simulink library "FG_Controller_Library"  (R2017b)
settings: Solver=VariableStepAuto  StartTime=0.0  StopTime=10.0  RelTol=1e-3
undefined symbols (not defined in the file or in its folder): fcut_velocity_joint, GaitLibrary, isSim, UserParams
libraries: slrtlib x113, simulink x1, func_block_library x1
(part 2 of 3)

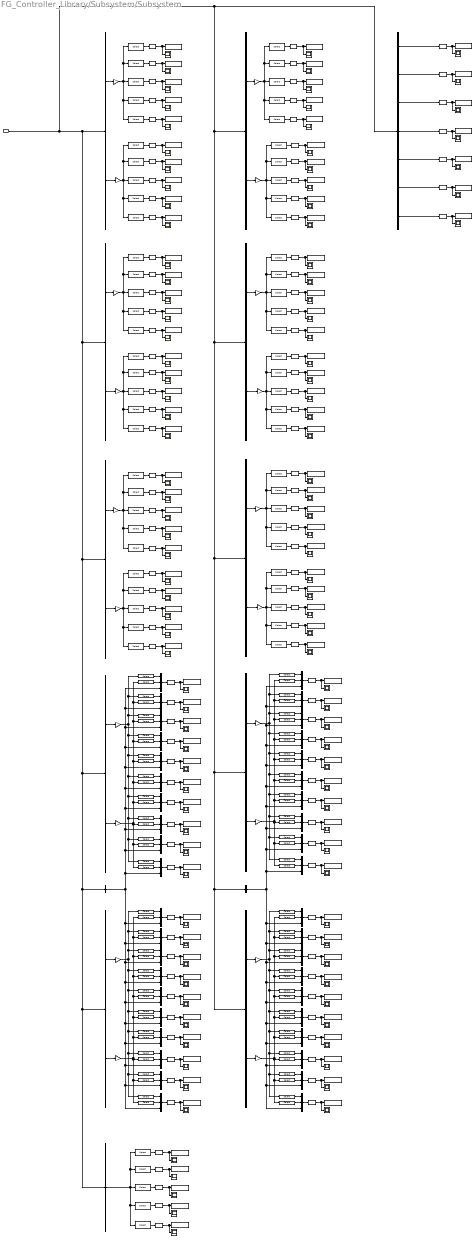
== system FG_Controller_Library/Subsystem/Subsystem ==
  In1 : Inport  OutDataTypeStr=Bus: cassieDataBus
  Bus Selector : BusSelector  OutputSignals=hd,dhd
  Bus Selector1 : BusSelector  OutputSignals=hd_joint,dhd_joint
  Bus Selector10 : BusSelector  OutputSignals=dh0_joint,dhd_joint
  Bus Selector11 : BusSelector  OutputSignals=stanceLeg
  Bus Selector12 : BusSelector  OutputSignals=u
  Bus Selector13 : BusSelector  OutputSignals=torso_vx_b,torso_vy_b,torso_vz_b,torso_vx_b_fil,torso_vy_b_fil,torso_vz_b_fil,tg_velocity_x
  Bus Selector2 : BusSelector  OutputSignals=h0,dh0
  Bus Selector3 : BusSelector  OutputSignals=h0_joint,dh0_joint
  Bus Selector4 : BusSelector  OutputSignals=y,dy
  Bus Selector5 : BusSelector  OutputSignals=y_joint,dy_joint
  Bus Selector6 : BusSelector  OutputSignals=hd,h0
  Bus Selector7 : BusSelector  OutputSignals=stanceLeg
  Bus Selector8 : BusSelector  OutputSignals=hd_joint,h0_joint
  Bus Selector9 : BusSelector  OutputSignals=dhd,dh0
  Gain{,1..19} (20 alike) : Gain  Gain=180/pi
  Mux{,1..39} (40 alike) : Mux  Inputs=3
  Reshape{,1..111} (112 alike) : Reshape
  Scope{,1..111} (112 alike) : Scope
  "Scope " : slrtlib/Displays and Logging/Scope   scopeno=201  scopetype=Host  autostart=on  viewmode=Graphical redraw  formatstr='%15.6f'  grid=on  ylimits=[0,0]  nosamples=2500  noprepostsamples=0  interleave=1  triggermode=FreeRun  triggersignal=1  trigsignalfromport=off  triggerlevel=0.0  triggerslope=Either  triggerscope=1  triggersample=0  filename=data.dat  mode=Lazy  writesize=512  autorestart=off  dynamicfilemode=off  maxwritefilesize=512*1024^2
  Scope 1 : slrtlib/Displays and Logging/Scope   scopeno=202  scopetype=Host  autostart=on  viewmode=Graphical redraw  formatstr='%15.6f'  grid=on  ylimits=[0,0]  nosamples=2500  noprepostsamples=0  interleave=1  triggermode=FreeRun  triggersignal=1  trigsignalfromport=off  triggerlevel=0.0  triggerslope=Either  triggerscope=1  triggersample=0  filename=data.dat  mode=Lazy  writesize=512  autorestart=off  dynamicfilemode=off  maxwritefilesize=512*1024^2
  Scope 10 : slrtlib/Displays and Logging/Scope   scopeno=2201  scopetype=Host  autostart=on  viewmode=Graphical redraw  formatstr='%15.6f'  grid=on  ylimits=[0,0]  nosamples=2500  noprepostsamples=0  interleave=1  triggermode=FreeRun  triggersignal=1  trigsignalfromport=off  triggerlevel=0.0  triggerslope=Either  triggerscope=1  triggersample=0  filename=data.dat  mode=Lazy  writesize=512  autorestart=off  dynamicfilemode=off  maxwritefilesize=512*1024^2
  Scope 100 : slrtlib/Displays and Logging/Scope   scopeno=701  scopetype=Host  autostart=on  viewmode=Graphical redraw  formatstr='%15.6f'  grid=on  ylimits=[0,0]  nosamples=2500  noprepostsamples=0  interleave=1  triggermode=FreeRun  triggersignal=1  trigsignalfromport=off  triggerlevel=0.0  triggerslope=Either  triggerscope=1  triggersample=0  filename=data.dat  mode=Lazy  writesize=512  autorestart=off  dynamicfilemode=off  maxwritefilesize=512*1024^2
  Scope 101 : slrtlib/Displays and Logging/Scope   scopeno=702  scopetype=Host  autostart=on  viewmode=Graphical redraw  formatstr='%15.6f'  grid=on  ylimits=[0,0]  nosamples=2500  noprepostsamples=0  interleave=1  triggermode=FreeRun  triggersignal=1  trigsignalfromport=off  triggerlevel=0.0  triggerslope=Either  triggerscope=1  triggersample=0  filename=data.dat  mode=Lazy  writesize=512  autorestart=off  dynamicfilemode=off  maxwritefilesize=512*1024^2
  Scope 102 : slrtlib/Displays and Logging/Scope   scopeno=703  scopetype=Host  autostart=on  viewmode=Graphical redraw  formatstr='%15.6f'  grid=on  ylimits=[0,0]  nosamples=2500  noprepostsamples=0  interleave=1  triggermode=FreeRun  triggersignal=1  trigsignalfromport=off  triggerlevel=0.0  triggerslope=Either  triggerscope=1  triggersample=0  filename=data.dat  mode=Lazy  writesize=512  autorestart=off  dynamicfilemode=off  maxwritefilesize=512*1024^2
  Scope 103 : slrtlib/Displays and Logging/Scope   scopeno=704  scopetype=Host  autostart=on  viewmode=Graphical redraw  formatstr='%15.6f'  grid=on  ylimits=[0,0]  nosamples=2500  noprepostsamples=0  interleave=1  triggermode=FreeRun  triggersignal=1  trigsignalfromport=off  triggerlevel=0.0  triggerslope=Either  triggerscope=1  triggersample=0  filename=data.dat  mode=Lazy  writesize=512  autorestart=off  dynamicfilemode=off  maxwritefilesize=512*1024^2
  Scope 104 : slrtlib/Displays and Logging/Scope   scopeno=705  scopetype=Host  autostart=on  viewmode=Graphical redraw  formatstr='%15.6f'  grid=on  ylimits=[0,0]  nosamples=2500  noprepostsamples=0  interleave=1  triggermode=FreeRun  triggersignal=1  trigsignalfromport=off  triggerlevel=0.0  triggerslope=Either  triggerscope=1  triggersample=0  filename=data.dat  mode=Lazy  writesize=512  autorestart=off  dynamicfilemode=off  maxwritefilesize=512*1024^2
  Scope 105 : slrtlib/Displays and Logging/Scope   scopeno=901  scopetype=Host  autostart=on  viewmode=Graphical redraw  formatstr='%15.6f'  grid=on  ylimits=[0,0]  nosamples=2500  noprepostsamples=0  interleave=1  triggermode=FreeRun  triggersignal=1  trigsignalfromport=off  triggerlevel=0.0  triggerslope=Either  triggerscope=1  triggersample=0  filename=data.dat  mode=Lazy  writesize=512  autorestart=off  dynamicfilemode=off  maxwritefilesize=512*1024^2
  Scope 106 : slrtlib/Displays and Logging/Scope   scopeno=902  scopetype=Host  autostart=on  viewmode=Graphical redraw  formatstr='%15.6f'  grid=on  ylimits=[0,0]  nosamples=2500  noprepostsamples=0  interleave=1  triggermode=FreeRun  triggersignal=1  trigsignalfromport=off  triggerlevel=0.0  triggerslope=Either  triggerscope=1  triggersample=0  filename=data.dat  mode=Lazy  writesize=512  autorestart=off  dynamicfilemode=off  maxwritefilesize=512*1024^2
  Scope 107 : slrtlib/Displays and Logging/Scope   scopeno=903  scopetype=Host  autostart=on  viewmode=Graphical redraw  formatstr='%15.6f'  grid=on  ylimits=[0,0]  nosamples=2500  noprepostsamples=0  interleave=1  triggermode=FreeRun  triggersignal=1  trigsignalfromport=off  triggerlevel=0.0  triggerslope=Either  triggerscope=1  triggersample=0  filename=data.dat  mode=Lazy  writesize=512  autorestart=off  dynamicfilemode=off  maxwritefilesize=512*1024^2
  Scope 108 : slrtlib/Displays and Logging/Scope   scopeno=904  scopetype=Host  autostart=on  viewmode=Graphical redraw  formatstr='%15.6f'  grid=on  ylimits=[0,0]  nosamples=2500  noprepostsamples=0  interleave=1  triggermode=FreeRun  triggersignal=1  trigsignalfromport=off  triggerlevel=0.0  triggerslope=Either  triggerscope=1  triggersample=0  filename=data.dat  mode=Lazy  writesize=512  autorestart=off  dynamicfilemode=off  maxwritefilesize=512*1024^2
  Scope 109 : slrtlib/Displays and Logging/Scope   scopeno=905  scopetype=Host  autostart=on  viewmode=Graphical redraw  formatstr='%15.6f'  grid=on  ylimits=[0,0]  nosamples=2500  noprepostsamples=0  interleave=1  triggermode=FreeRun  triggersignal=1  trigsignalfromport=off  triggerlevel=0.0  triggerslope=Either  triggerscope=1  triggersample=0  filename=data.dat  mode=Lazy  writesize=512  autorestart=off  dynamicfilemode=off  maxwritefilesize=512*1024^2
  Scope 11 : slrtlib/Displays and Logging/Scope   scopeno=2202  scopetype=Host  autostart=on  viewmode=Graphical redraw  formatstr='%15.6f'  grid=on  ylimits=[0,0]  nosamples=2500  noprepostsamples=0  interleave=1  triggermode=FreeRun  triggersignal=1  trigsignalfromport=off  triggerlevel=0.0  triggerslope=Either  triggerscope=1  triggersample=0  filename=data.dat  mode=Lazy  writesize=512  autorestart=off  dynamicfilemode=off  maxwritefilesize=512*1024^2
  Scope 110 : slrtlib/Displays and Logging/Scope   scopeno=906  scopetype=Host  autostart=on  viewmode=Graphical redraw  formatstr='%15.6f'  grid=on  ylimits=[0,0]  nosamples=2500  noprepostsamples=0  interleave=1  triggermode=FreeRun  triggersignal=1  trigsignalfromport=off  triggerlevel=0.0  triggerslope=Either  triggerscope=1  triggersample=0  filename=data.dat  mode=Lazy  writesize=512  autorestart=off  dynamicfilemode=off  maxwritefilesize=512*1024^2
  Scope 111 : slrtlib/Displays and Logging/Scope   scopeno=907  scopetype=Host  autostart=on  viewmode=Graphical redraw  formatstr='%15.6f'  grid=on  ylimits=[0,0]  nosamples=2500  noprepostsamples=0  interleave=1  triggermode=FreeRun  triggersignal=1  trigsignalfromport=off  triggerlevel=0.0  triggerslope=Either  triggerscope=1  triggersample=0  filename=data.dat  mode=Lazy  writesize=512  autorestart=off  dynamicfilemode=off  maxwritefilesize=512*1024^2
  Scope 12 : slrtlib/Displays and Logging/Scope   scopeno=2203  scopetype=Host  autostart=on  viewmode=Graphical redraw  formatstr='%15.6f'  grid=on  ylimits=[0,0]  nosamples=2500  noprepostsamples=0  interleave=1  triggermode=FreeRun  triggersignal=1  trigsignalfromport=off  triggerlevel=0.0  triggerslope=Either  triggerscope=1  triggersample=0  filename=data.dat  mode=Lazy  writesize=512  autorestart=off  dynamicfilemode=off  maxwritefilesize=512*1024^2
  Scope 13 : slrtlib/Displays and Logging/Scope   scopeno=2204  scopetype=Host  autostart=on  viewmode=Graphical redraw  formatstr='%15.6f'  grid=on  ylimits=[0,0]  nosamples=2500  noprepostsamples=0  interleave=1  triggermode=FreeRun  triggersignal=1  trigsignalfromport=off  triggerlevel=0.0  triggerslope=Either  triggerscope=1  triggersample=0  filename=data.dat  mode=Lazy  writesize=512  autorestart=off  dynamicfilemode=off  maxwritefilesize=512*1024^2
  Scope 14 : slrtlib/Displays and Logging/Scope   scopeno=2205  scopetype=Host  autostart=on  viewmode=Graphical redraw  formatstr='%15.6f'  grid=on  ylimits=[0,0]  nosamples=2500  noprepostsamples=0  interleave=1  triggermode=FreeRun  triggersignal=1  trigsignalfromport=off  triggerlevel=0.0  triggerslope=Either  triggerscope=1  triggersample=0  filename=data.dat  mode=Lazy  writesize=512  autorestart=off  dynamicfilemode=off  maxwritefilesize=512*1024^2
  Scope 15 : slrtlib/Displays and Logging/Scope   scopeno=2206  scopetype=Host  autostart=on  viewmode=Graphical redraw  formatstr='%15.6f'  grid=on  ylimits=[0,0]  nosamples=2500  noprepostsamples=0  interleave=1  triggermode=FreeRun  triggersignal=1  trigsignalfromport=off  triggerlevel=0.0  triggerslope=Either  triggerscope=1  triggersample=0  filename=data.dat  mode=Lazy  writesize=512  autorestart=off  dynamicfilemode=off  maxwritefilesize=512*1024^2
  Scope 16 : slrtlib/Displays and Logging/Scope   scopeno=2207  scopetype=Host  autostart=on  viewmode=Graphical redraw  formatstr='%15.6f'  grid=on  ylimits=[0,0]  nosamples=2500  noprepostsamples=0  interleave=1  triggermode=FreeRun  triggersignal=1  trigsignalfromport=off  triggerlevel=0.0  triggerslope=Either  triggerscope=1  triggersample=0  filename=data.dat  mode=Lazy  writesize=512  autorestart=off  dynamicfilemode=off  maxwritefilesize=512*1024^2
  Scope 17 : slrtlib/Displays and Logging/Scope   scopeno=2208  scopetype=Host  autostart=on  viewmode=Graphical redraw  formatstr='%15.6f'  grid=on  ylimits=[0,0]  nosamples=2500  noprepostsamples=0  interleave=1  triggermode=FreeRun  triggersignal=1  trigsignalfromport=off  triggerlevel=0.0  triggerslope=Either  triggerscope=1  triggersample=0  filename=data.dat  mode=Lazy  writesize=512  autorestart=off  dynamicfilemode=off  maxwritefilesize=512*1024^2
  Scope 18 : slrtlib/Displays and Logging/Scope   scopeno=2209  scopetype=Host  autostart=on  viewmode=Graphical redraw  formatstr='%15.6f'  grid=on  ylimits=[0,0]  nosamples=2500  noprepostsamples=0  interleave=1  triggermode=FreeRun  triggersignal=1  trigsignalfromport=off  triggerlevel=0.0  triggerslope=Either  triggerscope=1  triggersample=0  filename=data.dat  mode=Lazy  writesize=512  autorestart=off  dynamicfilemode=off  maxwritefilesize=512*1024^2
  Scope 19 : slrtlib/Displays and Logging/Scope   scopeno=2210  scopetype=Host  autostart=on  viewmode=Graphical redraw  formatstr='%15.6f'  grid=on  ylimits=[0,0]  nosamples=2500  noprepostsamples=0  interleave=1  triggermode=FreeRun  triggersignal=1  trigsignalfromport=off  triggerlevel=0.0  triggerslope=Either  triggerscope=1  triggersample=0  filename=data.dat  mode=Lazy  writesize=512  autorestart=off  dynamicfilemode=off  maxwritefilesize=512*1024^2
  Scope 2 : slrtlib/Displays and Logging/Scope   scopeno=203  scopetype=Host  autostart=on  viewmode=Graphical redraw  formatstr='%15.6f'  grid=on  ylimits=[0,0]  nosamples=2500  noprepostsamples=0  interleave=1  triggermode=FreeRun  triggersignal=1  trigsignalfromport=off  triggerlevel=0.0  triggerslope=Either  triggerscope=1  triggersample=0  filename=data.dat  mode=Lazy  writesize=512  autorestart=off  dynamicfilemode=off  maxwritefilesize=512*1024^2
  Scope 20 : slrtlib/Displays and Logging/Scope   scopeno=301  scopetype=Host  autostart=on  viewmode=Graphical redraw  formatstr='%15.6f'  grid=on  ylimits=[0,0]  nosamples=2500  noprepostsamples=0  interleave=1  triggermode=FreeRun  triggersignal=1  trigsignalfromport=off  triggerlevel=0.0  triggerslope=Either  triggerscope=1  triggersample=0  filename=data.dat  mode=Lazy  writesize=512  autorestart=off  dynamicfilemode=off  maxwritefilesize=512*1024^2
  Scope 21 : slrtlib/Displays and Logging/Scope   scopeno=302  scopetype=Host  autostart=on  viewmode=Graphical redraw  formatstr='%15.6f'  grid=on  ylimits=[0,0]  nosamples=2500  noprepostsamples=0  interleave=1  triggermode=FreeRun  triggersignal=1  trigsignalfromport=off  triggerlevel=0.0  triggerslope=Either  triggerscope=1  triggersample=0  filename=data.dat  mode=Lazy  writesize=512  autorestart=off  dynamicfilemode=off  maxwritefilesize=512*1024^2
  Scope 22 : slrtlib/Displays and Logging/Scope   scopeno=303  scopetype=Host  autostart=on  viewmode=Graphical redraw  formatstr='%15.6f'  grid=on  ylimits=[0,0]  nosamples=2500  noprepostsamples=0  interleave=1  triggermode=FreeRun  triggersignal=1  trigsignalfromport=off  triggerlevel=0.0  triggerslope=Either  triggerscope=1  triggersample=0  filename=data.dat  mode=Lazy  writesize=512  autorestart=off  dynamicfilemode=off  maxwritefilesize=512*1024^2
  Scope 23 : slrtlib/Displays and Logging/Scope   scopeno=304  scopetype=Host  autostart=on  viewmode=Graphical redraw  formatstr='%15.6f'  grid=on  ylimits=[0,0]  nosamples=2500  noprepostsamples=0  interleave=1  triggermode=FreeRun  triggersignal=1  trigsignalfromport=off  triggerlevel=0.0  triggerslope=Either  triggerscope=1  triggersample=0  filename=data.dat  mode=Lazy  writesize=512  autorestart=off  dynamicfilemode=off  maxwritefilesize=512*1024^2
  Scope 24 : slrtlib/Displays and Logging/Scope   scopeno=305  scopetype=Host  autostart=on  viewmode=Graphical redraw  formatstr='%15.6f'  grid=on  ylimits=[0,0]  nosamples=2500  noprepostsamples=0  interleave=1  triggermode=FreeRun  triggersignal=1  trigsignalfromport=off  triggerlevel=0.0  triggerslope=Either  triggerscope=1  triggersample=0  filename=data.dat  mode=Lazy  writesize=512  autorestart=off  dynamicfilemode=off  maxwritefilesize=512*1024^2
  Scope 25 : slrtlib/Displays and Logging/Scope   scopeno=306  scopetype=Host  autostart=on  viewmode=Graphical redraw  formatstr='%15.6f'  grid=on  ylimits=[0,0]  nosamples=2500  noprepostsamples=0  interleave=1  triggermode=FreeRun  triggersignal=1  trigsignalfromport=off  triggerlevel=0.0  triggerslope=Either  triggerscope=1  triggersample=0  filename=data.dat  mode=Lazy  writesize=512  autorestart=off  dynamicfilemode=off  maxwritefilesize=512*1024^2
  Scope 26 : slrtlib/Displays and Logging/Scope   scopeno=307  scopetype=Host  autostart=on  viewmode=Graphical redraw  formatstr='%15.6f'  grid=on  ylimits=[0,0]  nosamples=2500  noprepostsamples=0  interleave=1  triggermode=FreeRun  triggersignal=1  trigsignalfromport=off  triggerlevel=0.0  triggerslope=Either  triggerscope=1  triggersample=0  filename=data.dat  mode=Lazy  writesize=512  autorestart=off  dynamicfilemode=off  maxwritefilesize=512*1024^2
  Scope 27 : slrtlib/Displays and Logging/Scope   scopeno=308  scopetype=Host  autostart=on  viewmode=Graphical redraw  formatstr='%15.6f'  grid=on  ylimits=[0,0]  nosamples=2500  noprepostsamples=0  interleave=1  triggermode=FreeRun  triggersignal=1  trigsignalfromport=off  triggerlevel=0.0  triggerslope=Either  triggerscope=1  triggersample=0  filename=data.dat  mode=Lazy  writesize=512  autorestart=off  dynamicfilemode=off  maxwritefilesize=512*1024^2
  Scope 28 : slrtlib/Displays and Logging/Scope   scopeno=309  scopetype=Host  autostart=on  viewmode=Graphical redraw  formatstr='%15.6f'  grid=on  ylimits=[0,0]  nosamples=2500  noprepostsamples=0  interleave=1  triggermode=FreeRun  triggersignal=1  trigsignalfromport=off  triggerlevel=0.0  triggerslope=Either  triggerscope=1  triggersample=0  filename=data.dat  mode=Lazy  writesize=512  autorestart=off  dynamicfilemode=off  maxwritefilesize=512*1024^2
  Scope 29 : slrtlib/Displays and Logging/Scope   scopeno=310  scopetype=Host  autostart=on  viewmode=Graphical redraw  formatstr='%15.6f'  grid=on  ylimits=[0,0]  nosamples=2500  noprepostsamples=0  interleave=1  triggermode=FreeRun  triggersignal=1  trigsignalfromport=off  triggerlevel=0.0  triggerslope=Either  triggerscope=1  triggersample=0  filename=data.dat  mode=Lazy  writesize=512  autorestart=off  dynamicfilemode=off  maxwritefilesize=512*1024^2
  Scope 3 : slrtlib/Displays and Logging/Scope   scopeno=204  scopetype=Host  autostart=on  viewmode=Graphical redraw  formatstr='%15.6f'  grid=on  ylimits=[0,0]  nosamples=2500  noprepostsamples=0  interleave=1  triggermode=FreeRun  triggersignal=1  trigsignalfromport=off  triggerlevel=0.0  triggerslope=Either  triggerscope=1  triggersample=0  filename=data.dat  mode=Lazy  writesize=512  autorestart=off  dynamicfilemode=off  maxwritefilesize=512*1024^2
  Scope 30 : slrtlib/Displays and Logging/Scope   scopeno=3301  scopetype=Host  autostart=on  viewmode=Graphical redraw  formatstr='%15.6f'  grid=on  ylimits=[0,0]  nosamples=2500  noprepostsamples=0  interleave=1  triggermode=FreeRun  triggersignal=1  trigsignalfromport=off  triggerlevel=0.0  triggerslope=Either  triggerscope=1  triggersample=0  filename=data.dat  mode=Lazy  writesize=512  autorestart=off  dynamicfilemode=off  maxwritefilesize=512*1024^2
  Scope 31 : slrtlib/Displays and Logging/Scope   scopeno=3302  scopetype=Host  autostart=on  viewmode=Graphical redraw  formatstr='%15.6f'  grid=on  ylimits=[0,0]  nosamples=2500  noprepostsamples=0  interleave=1  triggermode=FreeRun  triggersignal=1  trigsignalfromport=off  triggerlevel=0.0  triggerslope=Either  triggerscope=1  triggersample=0  filename=data.dat  mode=Lazy  writesize=512  autorestart=off  dynamicfilemode=off  maxwritefilesize=512*1024^2
  Scope 32 : slrtlib/Displays and Logging/Scope   scopeno=3303  scopetype=Host  autostart=on  viewmode=Graphical redraw  formatstr='%15.6f'  grid=on  ylimits=[0,0]  nosamples=2500  noprepostsamples=0  interleave=1  triggermode=FreeRun  triggersignal=1  trigsignalfromport=off  triggerlevel=0.0  triggerslope=Either  triggerscope=1  triggersample=0  filename=data.dat  mode=Lazy  writesize=512  autorestart=off  dynamicfilemode=off  maxwritefilesize=512*1024^2
  Scope 33 : slrtlib/Displays and Logging/Scope   scopeno=3304  scopetype=Host  autostart=on  viewmode=Graphical redraw  formatstr='%15.6f'  grid=on  ylimits=[0,0]  nosamples=2500  noprepostsamples=0  interleave=1  triggermode=FreeRun  triggersignal=1  trigsignalfromport=off  triggerlevel=0.0  triggerslope=Either  triggerscope=1  triggersample=0  filename=data.dat  mode=Lazy  writesize=512  autorestart=off  dynamicfilemode=off  maxwritefilesize=512*1024^2
  Scope 34 : slrtlib/Displays and Logging/Scope   scopeno=3305  scopetype=Host  autostart=on  viewmode=Graphical redraw  formatstr='%15.6f'  grid=on  ylimits=[0,0]  nosamples=2500  noprepostsamples=0  interleave=1  triggermode=FreeRun  triggersignal=1  trigsignalfromport=off  triggerlevel=0.0  triggerslope=Either  triggerscope=1  triggersample=0  filename=data.dat  mode=Lazy  writesize=512  autorestart=off  dynamicfilemode=off  maxwritefilesize=512*1024^2
  Scope 35 : slrtlib/Displays and Logging/Scope   scopeno=3306  scopetype=Host  autostart=on  viewmode=Graphical redraw  formatstr='%15.6f'  grid=on  ylimits=[0,0]  nosamples=2500  noprepostsamples=0  interleave=1  triggermode=FreeRun  triggersignal=1  trigsignalfromport=off  triggerlevel=0.0  triggerslope=Either  triggerscope=1  triggersample=0  filename=data.dat  mode=Lazy  writesize=512  autorestart=off  dynamicfilemode=off  maxwritefilesize=512*1024^2
  Scope 36 : slrtlib/Displays and Logging/Scope   scopeno=3307  scopetype=Host  autostart=on  viewmode=Graphical redraw  formatstr='%15.6f'  grid=on  ylimits=[0,0]  nosamples=2500  noprepostsamples=0  interleave=1  triggermode=FreeRun  triggersignal=1  trigsignalfromport=off  triggerlevel=0.0  triggerslope=Either  triggerscope=1  triggersample=0  filename=data.dat  mode=Lazy  writesize=512  autorestart=off  dynamicfilemode=off  maxwritefilesize=512*1024^2
  Scope 37 : slrtlib/Displays and Logging/Scope   scopeno=3308  scopetype=Host  autostart=on  viewmode=Graphical redraw  formatstr='%15.6f'  grid=on  ylimits=[0,0]  nosamples=2500  noprepostsamples=0  interleave=1  triggermode=FreeRun  triggersignal=1  trigsignalfromport=off  triggerlevel=0.0  triggerslope=Either  triggerscope=1  triggersample=0  filename=data.dat  mode=Lazy  writesize=512  autorestart=off  dynamicfilemode=off  maxwritefilesize=512*1024^2
  Scope 38 : slrtlib/Displays and Logging/Scope   scopeno=3309  scopetype=Host  autostart=on  viewmode=Graphical redraw  formatstr='%15.6f'  grid=on  ylimits=[0,0]  nosamples=2500  noprepostsamples=0  interleave=1  triggermode=FreeRun  triggersignal=1  trigsignalfromport=off  triggerlevel=0.0  triggerslope=Either  triggerscope=1  triggersample=0  filename=data.dat  mode=Lazy  writesize=512  autorestart=off  dynamicfilemode=off  maxwritefilesize=512*1024^2
  Scope 39 : slrtlib/Displays and Logging/Scope   scopeno=3310  scopetype=Host  autostart=on  viewmode=Graphical redraw  formatstr='%15.6f'  grid=on  ylimits=[0,0]  nosamples=2500  noprepostsamples=0  interleave=1  triggermode=FreeRun  triggersignal=1  trigsignalfromport=off  triggerlevel=0.0  triggerslope=Either  triggerscope=1  triggersample=0  filename=data.dat  mode=Lazy  writesize=512  autorestart=off  dynamicfilemode=off  maxwritefilesize=512*1024^2
  Scope 4 : slrtlib/Displays and Logging/Scope   scopeno=205  scopetype=Host  autostart=on  viewmode=Graphical redraw  formatstr='%15.6f'  grid=on  ylimits=[0,0]  nosamples=2500  noprepostsamples=0  interleave=1  triggermode=FreeRun  triggersignal=1  trigsignalfromport=off  triggerlevel=0.0  triggerslope=Either  triggerscope=1  triggersample=0  filename=data.dat  mode=Lazy  writesize=512  autorestart=off  dynamicfilemode=off  maxwritefilesize=512*1024^2
  Scope 40 : slrtlib/Displays and Logging/Scope   scopeno=401  scopetype=Host  autostart=on  viewmode=Graphical redraw  formatstr='%15.6f'  grid=on  ylimits=[0,0]  nosamples=2500  noprepostsamples=0  interleave=1  triggermode=FreeRun  triggersignal=1  trigsignalfromport=off  triggerlevel=0.0  triggerslope=Either  triggerscope=1  triggersample=0  filename=data.dat  mode=Lazy  writesize=512  autorestart=off  dynamicfilemode=off  maxwritefilesize=512*1024^2
  Scope 41 : slrtlib/Displays and Logging/Scope   scopeno=402  scopetype=Host  autostart=on  viewmode=Graphical redraw  formatstr='%15.6f'  grid=on  ylimits=[0,0]  nosamples=2500  noprepostsamples=0  interleave=1  triggermode=FreeRun  triggersignal=1  trigsignalfromport=off  triggerlevel=0.0  triggerslope=Either  triggerscope=1  triggersample=0  filename=data.dat  mode=Lazy  writesize=512  autorestart=off  dynamicfilemode=off  maxwritefilesize=512*1024^2
  Scope 42 : slrtlib/Displays and Logging/Scope   scopeno=403  scopetype=Host  autostart=on  viewmode=Graphical redraw  formatstr='%15.6f'  grid=on  ylimits=[0,0]  nosamples=2500  noprepostsamples=0  interleave=1  triggermode=FreeRun  triggersignal=1  trigsignalfromport=off  triggerlevel=0.0  triggerslope=Either  triggerscope=1  triggersample=0  filename=data.dat  mode=Lazy  writesize=512  autorestart=off  dynamicfilemode=off  maxwritefilesize=512*1024^2
  Scope 43 : slrtlib/Displays and Logging/Scope   scopeno=404  scopetype=Host  autostart=on  viewmode=Graphical redraw  formatstr='%15.6f'  grid=on  ylimits=[0,0]  nosamples=2500  noprepostsamples=0  interleave=1  triggermode=FreeRun  triggersignal=1  trigsignalfromport=off  triggerlevel=0.0  triggerslope=Either  triggerscope=1  triggersample=0  filename=data.dat  mode=Lazy  writesize=512  autorestart=off  dynamicfilemode=off  maxwritefilesize=512*1024^2
  Scope 44 : slrtlib/Displays and Logging/Scope   scopeno=405  scopetype=Host  autostart=on  viewmode=Graphical redraw  formatstr='%15.6f'  grid=on  ylimits=[0,0]  nosamples=2500  noprepostsamples=0  interleave=1  triggermode=FreeRun  triggersignal=1  trigsignalfromport=off  triggerlevel=0.0  triggerslope=Either  triggerscope=1  triggersample=0  filename=data.dat  mode=Lazy  writesize=512  autorestart=off  dynamicfilemode=off  maxwritefilesize=512*1024^2
  Scope 45 : slrtlib/Displays and Logging/Scope   scopeno=406  scopetype=Host  autostart=on  viewmode=Graphical redraw  formatstr='%15.6f'  grid=on  ylimits=[0,0]  nosamples=2500  noprepostsamples=0  interleave=1  triggermode=FreeRun  triggersignal=1  trigsignalfromport=off  triggerlevel=0.0  triggerslope=Either  triggerscope=1  triggersample=0  filename=data.dat  mode=Lazy  writesize=512  autorestart=off  dynamicfilemode=off  maxwritefilesize=512*1024^2
  Scope 46 : slrtlib/Displays and Logging/Scope   scopeno=407  scopetype=Host  autostart=on  viewmode=Graphical redraw  formatstr='%15.6f'  grid=on  ylimits=[0,0]  nosamples=2500  noprepostsamples=0  interleave=1  triggermode=FreeRun  triggersignal=1  trigsignalfromport=off  triggerlevel=0.0  triggerslope=Either  triggerscope=1  triggersample=0  filename=data.dat  mode=Lazy  writesize=512  autorestart=off  dynamicfilemode=off  maxwritefilesize=512*1024^2
  Scope 47 : slrtlib/Displays and Logging/Scope   scopeno=408  scopetype=Host  autostart=on  viewmode=Graphical redraw  formatstr='%15.6f'  grid=on  ylimits=[0,0]  nosamples=2500  noprepostsamples=0  interleave=1  triggermode=FreeRun  triggersignal=1  trigsignalfromport=off  triggerlevel=0.0  triggerslope=Either  triggerscope=1  triggersample=0  filename=data.dat  mode=Lazy  writesize=512  autorestart=off  dynamicfilemode=off  maxwritefilesize=512*1024^2
  Scope 48 : slrtlib/Displays and Logging/Scope   scopeno=409  scopetype=Host  autostart=on  viewmode=Graphical redraw  formatstr='%15.6f'  grid=on  ylimits=[0,0]  nosamples=2500  noprepostsamples=0  interleave=1  triggermode=FreeRun  triggersignal=1  trigsignalfromport=off  triggerlevel=0.0  triggerslope=Either  triggerscope=1  triggersample=0  filename=data.dat  mode=Lazy  writesize=512  autorestart=off  dynamicfilemode=off  maxwritefilesize=512*1024^2
  Scope 49 : slrtlib/Displays and Logging/Scope   scopeno=410  scopetype=Host  autostart=on  viewmode=Graphical redraw  formatstr='%15.6f'  grid=on  ylimits=[0,0]  nosamples=2500  noprepostsamples=0  interleave=1  triggermode=FreeRun  triggersignal=1  trigsignalfromport=off  triggerlevel=0.0  triggerslope=Either  triggerscope=1  triggersample=0  filename=data.dat  mode=Lazy  writesize=512  autorestart=off  dynamicfilemode=off  maxwritefilesize=512*1024^2
  Scope 5 : slrtlib/Displays and Logging/Scope   scopeno=206  scopetype=Host  autostart=on  viewmode=Graphical redraw  formatstr='%15.6f'  grid=on  ylimits=[0,0]  nosamples=2500  noprepostsamples=0  interleave=1  triggermode=FreeRun  triggersignal=1  trigsignalfromport=off  triggerlevel=0.0  triggerslope=Either  triggerscope=1  triggersample=0  filename=data.dat  mode=Lazy  writesize=512  autorestart=off  dynamicfilemode=off  maxwritefilesize=512*1024^2
  Scope 50 : slrtlib/Displays and Logging/Scope   scopeno=4401  scopetype=Host  autostart=on  viewmode=Graphical redraw  formatstr='%15.6f'  grid=on  ylimits=[0,0]  nosamples=2500  noprepostsamples=0  interleave=1  triggermode=FreeRun  triggersignal=1  trigsignalfromport=off  triggerlevel=0.0  triggerslope=Either  triggerscope=1  triggersample=0  filename=data.dat  mode=Lazy  writesize=512  autorestart=off  dynamicfilemode=off  maxwritefilesize=512*1024^2
  Scope 51 : slrtlib/Displays and Logging/Scope   scopeno=4402  scopetype=Host  autostart=on  viewmode=Graphical redraw  formatstr='%15.6f'  grid=on  ylimits=[0,0]  nosamples=2500  noprepostsamples=0  interleave=1  triggermode=FreeRun  triggersignal=1  trigsignalfromport=off  triggerlevel=0.0  triggerslope=Either  triggerscope=1  triggersample=0  filename=data.dat  mode=Lazy  writesize=512  autorestart=off  dynamicfilemode=off  maxwritefilesize=512*1024^2
  Scope 52 : slrtlib/Displays and Logging/Scope   scopeno=4403  scopetype=Host  autostart=on  viewmode=Graphical redraw  formatstr='%15.6f'  grid=on  ylimits=[0,0]  nosamples=2500  noprepostsamples=0  interleave=1  triggermode=FreeRun  triggersignal=1  trigsignalfromport=off  triggerlevel=0.0  triggerslope=Either  triggerscope=1  triggersample=0  filename=data.dat  mode=Lazy  writesize=512  autorestart=off  dynamicfilemode=off  maxwritefilesize=512*1024^2
  Scope 53 : slrtlib/Displays and Logging/Scope   scopeno=4404  scopetype=Host  autostart=on  viewmode=Graphical redraw  formatstr='%15.6f'  grid=on  ylimits=[0,0]  nosamples=2500  noprepostsamples=0  interleave=1  triggermode=FreeRun  triggersignal=1  trigsignalfromport=off  triggerlevel=0.0  triggerslope=Either  triggerscope=1  triggersample=0  filename=data.dat  mode=Lazy  writesize=512  autorestart=off  dynamicfilemode=off  maxwritefilesize=512*1024^2
  Scope 54 : slrtlib/Displays and Logging/Scope   scopeno=4405  scopetype=Host  autostart=on  viewmode=Graphical redraw  formatstr='%15.6f'  grid=on  ylimits=[0,0]  nosamples=2500  noprepostsamples=0  interleave=1  triggermode=FreeRun  triggersignal=1  trigsignalfromport=off  triggerlevel=0.0  triggerslope=Either  triggerscope=1  triggersample=0  filename=data.dat  mode=Lazy  writesize=512  autorestart=off  dynamicfilemode=off  maxwritefilesize=512*1024^2
  Scope 55 : slrtlib/Displays and Logging/Scope   scopeno=4406  scopetype=Host  autostart=on  viewmode=Graphical redraw  formatstr='%15.6f'  grid=on  ylimits=[0,0]  nosamples=2500  noprepostsamples=0  interleave=1  triggermode=FreeRun  triggersignal=1  trigsignalfromport=off  triggerlevel=0.0  triggerslope=Either  triggerscope=1  triggersample=0  filename=data.dat  mode=Lazy  writesize=512  autorestart=off  dynamicfilemode=off  maxwritefilesize=512*1024^2
  Scope 56 : slrtlib/Displays and Logging/Scope   scopeno=4407  scopetype=Host  autostart=on  viewmode=Graphical redraw  formatstr='%15.6f'  grid=on  ylimits=[0,0]  nosamples=2500  noprepostsamples=0  interleave=1  triggermode=FreeRun  triggersignal=1  trigsignalfromport=off  triggerlevel=0.0  triggerslope=Either  triggerscope=1  triggersample=0  filename=data.dat  mode=Lazy  writesize=512  autorestart=off  dynamicfilemode=off  maxwritefilesize=512*1024^2
  Scope 57 : slrtlib/Displays and Logging/Scope   scopeno=4408  scopetype=Host  autostart=on  viewmode=Graphical redraw  formatstr='%15.6f'  grid=on  ylimits=[0,0]  nosamples=2500  noprepostsamples=0  interleave=1  triggermode=FreeRun  triggersignal=1  trigsignalfromport=off  triggerlevel=0.0  triggerslope=Either  triggerscope=1  triggersample=0  filename=data.dat  mode=Lazy  writesize=512  autorestart=off  dynamicfilemode=off  maxwritefilesize=512*1024^2
  Scope 58 : slrtlib/Displays and Logging/Scope   scopeno=4409  scopetype=Host  autostart=on  viewmode=Graphical redraw  formatstr='%15.6f'  grid=on  ylimits=[0,0]  nosamples=2500  noprepostsamples=0  interleave=1  triggermode=FreeRun  triggersignal=1  trigsignalfromport=off  triggerlevel=0.0  triggerslope=Either  triggerscope=1  triggersample=0  filename=data.dat  mode=Lazy  writesize=512  autorestart=off  dynamicfilemode=off  maxwritefilesize=512*1024^2
  Scope 59 : slrtlib/Displays and Logging/Scope   scopeno=4410  scopetype=Host  autostart=on  viewmode=Graphical redraw  formatstr='%15.6f'  grid=on  ylimits=[0,0]  nosamples=2500  noprepostsamples=0  interleave=1  triggermode=FreeRun  triggersignal=1  trigsignalfromport=off  triggerlevel=0.0  triggerslope=Either  triggerscope=1  triggersample=0  filename=data.dat  mode=Lazy  writesize=512  autorestart=off  dynamicfilemode=off  maxwritefilesize=512*1024^2
  Scope 6 : slrtlib/Displays and Logging/Scope   scopeno=207  scopetype=Host  autostart=on  viewmode=Graphical redraw  formatstr='%15.6f'  grid=on  ylimits=[0,0]  nosamples=2500  noprepostsamples=0  interleave=1  triggermode=FreeRun  triggersignal=1  trigsignalfromport=off  triggerlevel=0.0  triggerslope=Either  triggerscope=1  triggersample=0  filename=data.dat  mode=Lazy  writesize=512  autorestart=off  dynamicfilemode=off  maxwritefilesize=512*1024^2
  Scope 60 : slrtlib/Displays and Logging/Scope   scopeno=501  scopetype=Host  autostart=on  viewmode=Graphical redraw  formatstr='%15.6f'  grid=on  ylimits=[0,0]  nosamples=2500  noprepostsamples=0  interleave=1  triggermode=FreeRun  triggersignal=1  trigsignalfromport=off  triggerlevel=0.0  triggerslope=Either  triggerscope=1  triggersample=0  filename=data.dat  mode=Lazy  writesize=512  autorestart=off  dynamicfilemode=off  maxwritefilesize=512*1024^2
  Scope 61 : slrtlib/Displays and Logging/Scope   scopeno=502  scopetype=Host  autostart=on  viewmode=Graphical redraw  formatstr='%15.6f'  grid=on  ylimits=[0,0]  nosamples=2500  noprepostsamples=0  interleave=1  triggermode=FreeRun  triggersignal=1  trigsignalfromport=off  triggerlevel=0.0  triggerslope=Either  triggerscope=1  triggersample=0  filename=data.dat  mode=Lazy  writesize=512  autorestart=off  dynamicfilemode=off  maxwritefilesize=512*1024^2
  Scope 62 : slrtlib/Displays and Logging/Scope   scopeno=503  scopetype=Host  autostart=on  viewmode=Graphical redraw  formatstr='%15.6f'  grid=on  ylimits=[0,0]  nosamples=2500  noprepostsamples=0  interleave=1  triggermode=FreeRun  triggersignal=1  trigsignalfromport=off  triggerlevel=0.0  triggerslope=Either  triggerscope=1  triggersample=0  filename=data.dat  mode=Lazy  writesize=512  autorestart=off  dynamicfilemode=off  maxwritefilesize=512*1024^2
  Scope 63 : slrtlib/Displays and Logging/Scope   scopeno=504  scopetype=Host  autostart=on  viewmode=Graphical redraw  formatstr='%15.6f'  grid=on  ylimits=[0,0]  nosamples=2500  noprepostsamples=0  interleave=1  triggermode=FreeRun  triggersignal=1  trigsignalfromport=off  triggerlevel=0.0  triggerslope=Either  triggerscope=1  triggersample=0  filename=data.dat  mode=Lazy  writesize=512  autorestart=off  dynamicfilemode=off  maxwritefilesize=512*1024^2
  Scope 64 : slrtlib/Displays and Logging/Scope   scopeno=505  scopetype=Host  autostart=on  viewmode=Graphical redraw  formatstr='%15.6f'  grid=on  ylimits=[0,0]  nosamples=2500  noprepostsamples=0  interleave=1  triggermode=FreeRun  triggersignal=1  trigsignalfromport=off  triggerlevel=0.0  triggerslope=Either  triggerscope=1  triggersample=0  filename=data.dat  mode=Lazy  writesize=512  autorestart=off  dynamicfilemode=off  maxwritefilesize=512*1024^2
  Scope 65 : slrtlib/Displays and Logging/Scope   scopeno=506  scopetype=Host  autostart=on  viewmode=Graphical redraw  formatstr='%15.6f'  grid=on  ylimits=[0,0]  nosamples=2500  noprepostsamples=0  interleave=1  triggermode=FreeRun  triggersignal=1  trigsignalfromport=off  triggerlevel=0.0  triggerslope=Either  triggerscope=1  triggersample=0  filename=data.dat  mode=Lazy  writesize=512  autorestart=off  dynamicfilemode=off  maxwritefilesize=512*1024^2
  Scope 66 : slrtlib/Displays and Logging/Scope   scopeno=507  scopetype=Host  autostart=on  viewmode=Graphical redraw  formatstr='%15.6f'  grid=on  ylimits=[0,0]  nosamples=2500  noprepostsamples=0  interleave=1  triggermode=FreeRun  triggersignal=1  trigsignalfromport=off  triggerlevel=0.0  triggerslope=Either  triggerscope=1  triggersample=0  filename=data.dat  mode=Lazy  writesize=512  autorestart=off  dynamicfilemode=off  maxwritefilesize=512*1024^2
  Scope 67 : slrtlib/Displays and Logging/Scope   scopeno=508  scopetype=Host  autostart=on  viewmode=Graphical redraw  formatstr='%15.6f'  grid=on  ylimits=[0,0]  nosamples=2500  noprepostsamples=0  interleave=1  triggermode=FreeRun  triggersignal=1  trigsignalfromport=off  triggerlevel=0.0  triggerslope=Either  triggerscope=1  triggersample=0  filename=data.dat  mode=Lazy  writesize=512  autorestart=off  dynamicfilemode=off  maxwritefilesize=512*1024^2
  Scope 68 : slrtlib/Displays and Logging/Scope   scopeno=509  scopetype=Host  autostart=on  viewmode=Graphical redraw  formatstr='%15.6f'  grid=on  ylimits=[0,0]  nosamples=2500  noprepostsamples=0  interleave=1  triggermode=FreeRun  triggersignal=1  trigsignalfromport=off  triggerlevel=0.0  triggerslope=Either  triggerscope=1  triggersample=0  filename=data.dat  mode=Lazy  writesize=512  autorestart=off  dynamicfilemode=off  maxwritefilesize=512*1024^2
  Scope 69 : slrtlib/Displays and Logging/Scope   scopeno=510  scopetype=Host  autostart=on  viewmode=Graphical redraw  formatstr='%15.6f'  grid=on  ylimits=[0,0]  nosamples=2500  noprepostsamples=0  interleave=1  triggermode=FreeRun  triggersignal=1  trigsignalfromport=off  triggerlevel=0.0  triggerslope=Either  triggerscope=1  triggersample=0  filename=data.dat  mode=Lazy  writesize=512  autorestart=off  dynamicfilemode=off  maxwritefilesize=512*1024^2
  Scope 7 : slrtlib/Displays and Logging/Scope   scopeno=208  scopetype=Host  autostart=on  viewmode=Graphical redraw  formatstr='%15.6f'  grid=on  ylimits=[0,0]  nosamples=2500  noprepostsamples=0  interleave=1  triggermode=FreeRun  triggersignal=1  trigsignalfromport=off  triggerlevel=0.0  triggerslope=Either  triggerscope=1  triggersample=0  filename=data.dat  mode=Lazy  writesize=512  autorestart=off  dynamicfilemode=off  maxwritefilesize=512*1024^2
  Scope 70 : slrtlib/Displays and Logging/Scope   scopeno=5501  scopetype=Host  autostart=on  viewmode=Graphical redraw  formatstr='%15.6f'  grid=on  ylimits=[0,0]  nosamples=2500  noprepostsamples=0  interleave=1  triggermode=FreeRun  triggersignal=1  trigsignalfromport=off  triggerlevel=0.0  triggerslope=Either  triggerscope=1  triggersample=0  filename=data.dat  mode=Lazy  writesize=512  autorestart=off  dynamicfilemode=off  maxwritefilesize=512*1024^2
  Scope 71 : slrtlib/Displays and Logging/Scope   scopeno=5502  scopetype=Host  autostart=on  viewmode=Graphical redraw  formatstr='%15.6f'  grid=on  ylimits=[0,0]  nosamples=2500  noprepostsamples=0  interleave=1  triggermode=FreeRun  triggersignal=1  trigsignalfromport=off  triggerlevel=0.0  triggerslope=Either  triggerscope=1  triggersample=0  filename=data.dat  mode=Lazy  writesize=512  autorestart=off  dynamicfilemode=off  maxwritefilesize=512*1024^2
  Scope 72 : slrtlib/Displays and Logging/Scope   scopeno=5503  scopetype=Host  autostart=on  viewmode=Graphical redraw  formatstr='%15.6f'  grid=on  ylimits=[0,0]  nosamples=2500  noprepostsamples=0  interleave=1  triggermode=FreeRun  triggersignal=1  trigsignalfromport=off  triggerlevel=0.0  triggerslope=Either  triggerscope=1  triggersample=0  filename=data.dat  mode=Lazy  writesize=512  autorestart=off  dynamicfilemode=off  maxwritefilesize=512*1024^2
  Scope 73 : slrtlib/Displays and Logging/Scope   scopeno=5504  scopetype=Host  autostart=on  viewmode=Graphical redraw  formatstr='%15.6f'  grid=on  ylimits=[0,0]  nosamples=2500  noprepostsamples=0  interleave=1  triggermode=FreeRun  triggersignal=1  trigsignalfromport=off  triggerlevel=0.0  triggerslope=Either  triggerscope=1  triggersample=0  filename=data.dat  mode=Lazy  writesize=512  autorestart=off  dynamicfilemode=off  maxwritefilesize=512*1024^2
  Scope 74 : slrtlib/Displays and Logging/Scope   scopeno=5505  scopetype=Host  autostart=on  viewmode=Graphical redraw  formatstr='%15.6f'  grid=on  ylimits=[0,0]  nosamples=2500  noprepostsamples=0  interleave=1  triggermode=FreeRun  triggersignal=1  trigsignalfromport=off  triggerlevel=0.0  triggerslope=Either  triggerscope=1  triggersample=0  filename=data.dat  mode=Lazy  writesize=512  autorestart=off  dynamicfilemode=off  maxwritefilesize=512*1024^2
  Scope 75 : slrtlib/Displays and Logging/Scope   scopeno=5506  scopetype=Host  autostart=on  viewmode=Graphical redraw  formatstr='%15.6f'  grid=on  ylimits=[0,0]  nosamples=2500  noprepostsamples=0  interleave=1  triggermode=FreeRun  triggersignal=1  trigsignalfromport=off  triggerlevel=0.0  triggerslope=Either  triggerscope=1  triggersample=0  filename=data.dat  mode=Lazy  writesize=512  autorestart=off  dynamicfilemode=off  maxwritefilesize=512*1024^2
  Scope 76 : slrtlib/Displays and Logging/Scope   scopeno=5507  scopetype=Host  autostart=on  viewmode=Graphical redraw  formatstr='%15.6f'  grid=on  ylimits=[0,0]  nosamples=2500  noprepostsamples=0  interleave=1  triggermode=FreeRun  triggersignal=1  trigsignalfromport=off  triggerlevel=0.0  triggerslope=Either  triggerscope=1  triggersample=0  filename=data.dat  mode=Lazy  writesize=512  autorestart=off  dynamicfilemode=off  maxwritefilesize=512*1024^2
  Scope 77 : slrtlib/Displays and Logging/Scope   scopeno=5508  scopetype=Host  autostart=on  viewmode=Graphical redraw  formatstr='%15.6f'  grid=on  ylimits=[0,0]  nosamples=2500  noprepostsamples=0  interleave=1  triggermode=FreeRun  triggersignal=1  trigsignalfromport=off  triggerlevel=0.0  triggerslope=Either  triggerscope=1  triggersample=0  filename=data.dat  mode=Lazy  writesize=512  autorestart=off  dynamicfilemode=off  maxwritefilesize=512*1024^2
  Scope 78 : slrtlib/Displays and Logging/Scope   scopeno=5509  scopetype=Host  autostart=on  viewmode=Graphical redraw  formatstr='%15.6f'  grid=on  ylimits=[0,0]  nosamples=2500  noprepostsamples=0  interleave=1  triggermode=FreeRun  triggersignal=1  trigsignalfromport=off  triggerlevel=0.0  triggerslope=Either  triggerscope=1  triggersample=0  filename=data.dat  mode=Lazy  writesize=512  autorestart=off  dynamicfilemode=off  maxwritefilesize=512*1024^2
  Scope 79 : slrtlib/Displays and Logging/Scope   scopeno=5510  scopetype=Host  autostart=on  viewmode=Graphical redraw  formatstr='%15.6f'  grid=on  ylimits=[0,0]  nosamples=2500  noprepostsamples=0  interleave=1  triggermode=FreeRun  triggersignal=1  trigsignalfromport=off  triggerlevel=0.0  triggerslope=Either  triggerscope=1  triggersample=0  filename=data.dat  mode=Lazy  writesize=512  autorestart=off  dynamicfilemode=off  maxwritefilesize=512*1024^2
  Scope 8 : slrtlib/Displays and Logging/Scope   scopeno=209  scopetype=Host  autostart=on  viewmode=Graphical redraw  formatstr='%15.6f'  grid=on  ylimits=[0,0]  nosamples=2500  noprepostsamples=0  interleave=1  triggermode=FreeRun  triggersignal=1  trigsignalfromport=off  triggerlevel=0.0  triggerslope=Either  triggerscope=1  triggersample=0  filename=data.dat  mode=Lazy  writesize=512  autorestart=off  dynamicfilemode=off  maxwritefilesize=512*1024^2
  Scope 80 : slrtlib/Displays and Logging/Scope   scopeno=601  scopetype=Host  autostart=on  viewmode=Graphical redraw  formatstr='%15.6f'  grid=on  ylimits=[0,0]  nosamples=2500  noprepostsamples=0  interleave=1  triggermode=FreeRun  triggersignal=1  trigsignalfromport=off  triggerlevel=0.0  triggerslope=Either  triggerscope=1  triggersample=0  filename=data.dat  mode=Lazy  writesize=512  autorestart=off  dynamicfilemode=off  maxwritefilesize=512*1024^2
  Scope 81 : slrtlib/Displays and Logging/Scope   scopeno=602  scopetype=Host  autostart=on  viewmode=Graphical redraw  formatstr='%15.6f'  grid=on  ylimits=[0,0]  nosamples=2500  noprepostsamples=0  interleave=1  triggermode=FreeRun  triggersignal=1  trigsignalfromport=off  triggerlevel=0.0  triggerslope=Either  triggerscope=1  triggersample=0  filename=data.dat  mode=Lazy  writesize=512  autorestart=off  dynamicfilemode=off  maxwritefilesize=512*1024^2
  Scope 82 : slrtlib/Displays and Logging/Scope   scopeno=603  scopetype=Host  autostart=on  viewmode=Graphical redraw  formatstr='%15.6f'  grid=on  ylimits=[0,0]  nosamples=2500  noprepostsamples=0  interleave=1  triggermode=FreeRun  triggersignal=1  trigsignalfromport=off  triggerlevel=0.0  triggerslope=Either  triggerscope=1  triggersample=0  filename=data.dat  mode=Lazy  writesize=512  autorestart=off  dynamicfilemode=off  maxwritefilesize=512*1024^2
  Scope 83 : slrtlib/Displays and Logging/Scope   scopeno=604  scopetype=Host  autostart=on  viewmode=Graphical redraw  formatstr='%15.6f'  grid=on  ylimits=[0,0]  nosamples=2500  noprepostsamples=0  interleave=1  triggermode=FreeRun  triggersignal=1  trigsignalfromport=off  triggerlevel=0.0  triggerslope=Either  triggerscope=1  triggersample=0  filename=data.dat  mode=Lazy  writesize=512  autorestart=off  dynamicfilemode=off  maxwritefilesize=512*1024^2
  Scope 84 : slrtlib/Displays and Logging/Scope   scopeno=605  scopetype=Host  autostart=on  viewmode=Graphical redraw  formatstr='%15.6f'  grid=on  ylimits=[0,0]  nosamples=2500  noprepostsamples=0  interleave=1  triggermode=FreeRun  triggersignal=1  trigsignalfromport=off  triggerlevel=0.0  triggerslope=Either  triggerscope=1  triggersample=0  filename=data.dat  mode=Lazy  writesize=512  autorestart=off  dynamicfilemode=off  maxwritefilesize=512*1024^2
  Scope 85 : slrtlib/Displays and Logging/Scope   scopeno=606  scopetype=Host  autostart=on  viewmode=Graphical redraw  formatstr='%15.6f'  grid=on  ylimits=[0,0]  nosamples=2500  noprepostsamples=0  interleave=1  triggermode=FreeRun  triggersignal=1  trigsignalfromport=off  triggerlevel=0.0  triggerslope=Either  triggerscope=1  triggersample=0  filename=data.dat  mode=Lazy  writesize=512  autorestart=off  dynamicfilemode=off  maxwritefilesize=512*1024^2
  Scope 86 : slrtlib/Displays and Logging/Scope   scopeno=607  scopetype=Host  autostart=on  viewmode=Graphical redraw  formatstr='%15.6f'  grid=on  ylimits=[0,0]  nosamples=2500  noprepostsamples=0  interleave=1  triggermode=FreeRun  triggersignal=1  trigsignalfromport=off  triggerlevel=0.0  triggerslope=Either  triggerscope=1  triggersample=0  filename=data.dat  mode=Lazy  writesize=512  autorestart=off  dynamicfilemode=off  maxwritefilesize=512*1024^2
  Scope 87 : slrtlib/Displays and Logging/Scope   scopeno=608  scopetype=Host  autostart=on  viewmode=Graphical redraw  formatstr='%15.6f'  grid=on  ylimits=[0,0]  nosamples=2500  noprepostsamples=0  interleave=1  triggermode=FreeRun  triggersignal=1  trigsignalfromport=off  triggerlevel=0.0  triggerslope=Either  triggerscope=1  triggersample=0  filename=data.dat  mode=Lazy  writesize=512  autorestart=off  dynamicfilemode=off  maxwritefilesize=512*1024^2
  Scope 88 : slrtlib/Displays and Logging/Scope   scopeno=609  scopetype=Host  autostart=on  viewmode=Graphical redraw  formatstr='%15.6f'  grid=on  ylimits=[0,0]  nosamples=2500  noprepostsamples=0  interleave=1  triggermode=FreeRun  triggersignal=1  trigsignalfromport=off  triggerlevel=0.0  triggerslope=Either  triggerscope=1  triggersample=0  filename=data.dat  mode=Lazy  writesize=512  autorestart=off  dynamicfilemode=off  maxwritefilesize=512*1024^2
  Scope 89 : slrtlib/Displays and Logging/Scope   scopeno=610  scopetype=Host  autostart=on  viewmode=Graphical redraw  formatstr='%15.6f'  grid=on  ylimits=[0,0]  nosamples=2500  noprepostsamples=0  interleave=1  triggermode=FreeRun  triggersignal=1  trigsignalfromport=off  triggerlevel=0.0  triggerslope=Either  triggerscope=1  triggersample=0  filename=data.dat  mode=Lazy  writesize=512  autorestart=off  dynamicfilemode=off  maxwritefilesize=512*1024^2
  Scope 9 : slrtlib/Displays and Logging/Scope   scopeno=210  scopetype=Host  autostart=on  viewmode=Graphical redraw  formatstr='%15.6f'  grid=on  ylimits=[0,0]  nosamples=2500  noprepostsamples=0  interleave=1  triggermode=FreeRun  triggersignal=1  trigsignalfromport=off  triggerlevel=0.0  triggerslope=Either  triggerscope=1  triggersample=0  filename=data.dat  mode=Lazy  writesize=512  autorestart=off  dynamicfilemode=off  maxwritefilesize=512*1024^2
  Scope 90 : slrtlib/Displays and Logging/Scope   scopeno=6601  scopetype=Host  autostart=on  viewmode=Graphical redraw  formatstr='%15.6f'  grid=on  ylimits=[0,0]  nosamples=2500  noprepostsamples=0  interleave=1  triggermode=FreeRun  triggersignal=1  trigsignalfromport=off  triggerlevel=0.0  triggerslope=Either  triggerscope=1  triggersample=0  filename=data.dat  mode=Lazy  writesize=512  autorestart=off  dynamicfilemode=off  maxwritefilesize=512*1024^2
  Scope 91 : slrtlib/Displays and Logging/Scope   scopeno=6602  scopetype=Host  autostart=on  viewmode=Graphical redraw  formatstr='%15.6f'  grid=on  ylimits=[0,0]  nosamples=2500  noprepostsamples=0  interleave=1  triggermode=FreeRun  triggersignal=1  trigsignalfromport=off  triggerlevel=0.0  triggerslope=Either  triggerscope=1  triggersample=0  filename=data.dat  mode=Lazy  writesize=512  autorestart=off  dynamicfilemode=off  maxwritefilesize=512*1024^2
  Scope 92 : slrtlib/Displays and Logging/Scope   scopeno=6603  scopetype=Host  autostart=on  viewmode=Graphical redraw  formatstr='%15.6f'  grid=on  ylimits=[0,0]  nosamples=2500  noprepostsamples=0  interleave=1  triggermode=FreeRun  triggersignal=1  trigsignalfromport=off  triggerlevel=0.0  triggerslope=Either  triggerscope=1  triggersample=0  filename=data.dat  mode=Lazy  writesize=512  autorestart=off  dynamicfilemode=off  maxwritefilesize=512*1024^2
  Scope 93 : slrtlib/Displays and Logging/Scope   scopeno=6604  scopetype=Host  autostart=on  viewmode=Graphical redraw  formatstr='%15.6f'  grid=on  ylimits=[0,0]  nosamples=2500  noprepostsamples=0  interleave=1  triggermode=FreeRun  triggersignal=1  trigsignalfromport=off  triggerlevel=0.0  triggerslope=Either  triggerscope=1  triggersample=0  filename=data.dat  mode=Lazy  writesize=512  autorestart=off  dynamicfilemode=off  maxwritefilesize=512*1024^2
  Scope 94 : slrtlib/Displays and Logging/Scope   scopeno=6605  scopetype=Host  autostart=on  viewmode=Graphical redraw  formatstr='%15.6f'  grid=on  ylimits=[0,0]  nosamples=2500  noprepostsamples=0  interleave=1  triggermode=FreeRun  triggersignal=1  trigsignalfromport=off  triggerlevel=0.0  triggerslope=Either  triggerscope=1  triggersample=0  filename=data.dat  mode=Lazy  writesize=512  autorestart=off  dynamicfilemode=off  maxwritefilesize=512*1024^2
  Scope 95 : slrtlib/Displays and Logging/Scope   scopeno=6606  scopetype=Host  autostart=on  viewmode=Graphical redraw  formatstr='%15.6f'  grid=on  ylimits=[0,0]  nosamples=2500  noprepostsamples=0  interleave=1  triggermode=FreeRun  triggersignal=1  trigsignalfromport=off  triggerlevel=0.0  triggerslope=Either  triggerscope=1  triggersample=0  filename=data.dat  mode=Lazy  writesize=512  autorestart=off  dynamicfilemode=off  maxwritefilesize=512*1024^2
  Scope 96 : slrtlib/Displays and Logging/Scope   scopeno=6607  scopetype=Host  autostart=on  viewmode=Graphical redraw  formatstr='%15.6f'  grid=on  ylimits=[0,0]  nosamples=2500  noprepostsamples=0  interleave=1  triggermode=FreeRun  triggersignal=1  trigsignalfromport=off  triggerlevel=0.0  triggerslope=Either  triggerscope=1  triggersample=0  filename=data.dat  mode=Lazy  writesize=512  autorestart=off  dynamicfilemode=off  maxwritefilesize=512*1024^2
  Scope 97 : slrtlib/Displays and Logging/Scope   scopeno=6608  scopetype=Host  autostart=on  viewmode=Graphical redraw  formatstr='%15.6f'  grid=on  ylimits=[0,0]  nosamples=2500  noprepostsamples=0  interleave=1  triggermode=FreeRun  triggersignal=1  trigsignalfromport=off  triggerlevel=0.0  triggerslope=Either  triggerscope=1  triggersample=0  filename=data.dat  mode=Lazy  writesize=512  autorestart=off  dynamicfilemode=off  maxwritefilesize=512*1024^2
  Scope 98 : slrtlib/Displays and Logging/Scope   scopeno=6609  scopetype=Host  autostart=on  viewmode=Graphical redraw  formatstr='%15.6f'  grid=on  ylimits=[0,0]  nosamples=2500  noprepostsamples=0  interleave=1  triggermode=FreeRun  triggersignal=1  trigsignalfromport=off  triggerlevel=0.0  triggerslope=Either  triggerscope=1  triggersample=0  filename=data.dat  mode=Lazy  writesize=512  autorestart=off  dynamicfilemode=off  maxwritefilesize=512*1024^2
  Scope 99 : slrtlib/Displays and Logging/Scope   scopeno=6610  scopetype=Host  autostart=on  viewmode=Graphical redraw  formatstr='%15.6f'  grid=on  ylimits=[0,0]  nosamples=2500  noprepostsamples=0  interleave=1  triggermode=FreeRun  triggersignal=1  trigsignalfromport=off  triggerlevel=0.0  triggerslope=Either  triggerscope=1  triggersample=0  filename=data.dat  mode=Lazy  writesize=512  autorestart=off  dynamicfilemode=off  maxwritefilesize=512*1024^2
  Selector{,5,10,15,20,25,30,35,40,45,50,55,140} (13 alike) : Selector  InputPortWidth=10  IndexOptions=Index vector (dialog)  Indices=[1 6]  OutputSizes=1
  Selector{1,6,11,16,21,26,31,36,41,46,51,56,141} (13 alike) : Selector  InputPortWidth=10  IndexOptions=Index vector (dialog)  Indices=[2 7]  OutputSizes=1
  Selector{60,70,80,90,100,110,120,130} (8 alike) : Selector  InputPortWidth=10  IndexOptions=Index vector (dialog)  Indices=[1]  OutputSizes=1
  Selector{61,71,81,91,101,111,121,131} (8 alike) : Selector  InputPortWidth=10  IndexOptions=Index vector (dialog)  Indices=[2]  OutputSizes=1
  Selector{62,72,82,92,102,112,122,132} (8 alike) : Selector  InputPortWidth=10  IndexOptions=Index vector (dialog)  Indices=[3]  OutputSizes=1
  Selector{63,73,83,93,103,113,123,133} (8 alike) : Selector  InputPortWidth=10  IndexOptions=Index vector (dialog)  Indices=[4]  OutputSizes=1
  Selector{64,74,84,94,104,114,124,134} (8 alike) : Selector  InputPortWidth=10  IndexOptions=Index vector (dialog)  Indices=[5]  OutputSizes=1
  Selector{65,75,85,95,105,115,125,135} (8 alike) : Selector  InputPortWidth=10  IndexOptions=Index vector (dialog)  Indices=[6]  OutputSizes=1
  Selector{66,76,86,96,106,116,126,136} (8 alike) : Selector  InputPortWidth=10  IndexOptions=Index vector (dialog)  Indices=[7]  OutputSizes=1
  Selector{67,77,87,97,107,117,127,137} (8 alike) : Selector  InputPortWidth=10  IndexOptions=Index vector (dialog)  Indices=[8]  OutputSizes=1
  Selector{68,78,88,98,108,118,128,138} (8 alike) : Selector  InputPortWidth=10  IndexOptions=Index vector (dialog)  Indices=[9]  OutputSizes=1
  Selector{69,79,89,99,109,119,129,139} (8 alike) : Selector  InputPortWidth=10  IndexOptions=Index vector (dialog)  Indices=[10]  OutputSizes=1
  Selector{2,7,12,17,22,27,32,37,42,47,52,57,142} (13 alike) : Selector  InputPortWidth=10  IndexOptions=Index vector (dialog)  Indices=[3 8]  OutputSizes=1
  Selector{3,8,13,18,23,28,33,38,43,48,53,58,143} (13 alike) : Selector  InputPortWidth=10  IndexOptions=Index vector (dialog)  Indices=[4 9]  OutputSizes=1
  Selector{4,9,14,19,24,29,34,39,44,49,54,59,144} (13 alike) : Selector  InputPortWidth=10  IndexOptions=Index vector (dialog)  Indices=[5 10]  OutputSizes=1
  wires:
  Bus Selector/1 -> Gain/1  "<hd>"
  Gain/1 -> Selector4/1, Selector3/1, Selector2/1, Selector/1, Selector1/1
  Selector/1 -> Reshape/1
  Selector4/1 -> Reshape4/1
  Selector3/1 -> Reshape3/1
  Selector2/1 -> Reshape2/1
  Selector1/1 -> Reshape1/1
  Reshape/1 -> Scope/1, "Scope "/1
  Reshape1/1 -> Scope1/1, Scope 1/1
  Reshape2/1 -> Scope2/1, Scope 2/1
  Reshape3/1 -> Scope3/1, Scope 3/1
  Reshape4/1 -> Scope4/1, Scope 4/1
  Reshape6/1 -> Scope6/1, Scope 6/1
  Gain1/1 -> Selector9/1, Selector8/1, Selector7/1, Selector5/1, Selector6/1
  Reshape8/1 -> Scope8/1, Scope 8/1
  Selector6/1 -> Reshape6/1
  Selector7/1 -> Reshape7/1
  Bus Selector/2 -> Gain1/1  "<dhd>"
  Selector5/1 -> Reshape5/1
  Reshape5/1 -> Scope5/1, Scope 5/1
  Selector9/1 -> Reshape9/1
  Reshape9/1 -> Scope9/1, Scope 9/1
  Reshape7/1 -> Scope7/1, Scope 7/1
  Selector8/1 -> Reshape8/1
  Gain2/1 -> Selector14/1, Selector13/1, Selector12/1, Selector10/1, Selector11/1
  Reshape13/1 -> Scope13/1, Scope 13/1
  Bus Selector1/2 -> Gain3/1  "<dhd_joint>"
  Selector12/1 -> Reshape12/1
  Reshape19/1 -> Scope19/1, Scope 19/1
  Selector19/1 -> Reshape19/1
  Bus Selector1/1 -> Gain2/1  "<hd_joint>"
  Reshape15/1 -> Scope15/1, Scope 15/1
  Selector15/1 -> Reshape15/1
  Gain3/1 -> Selector19/1, Selector18/1, Selector17/1, Selector15/1, Selector16/1
  Selector17/1 -> Reshape17/1
  Reshape18/1 -> Scope18/1, Scope 18/1
  Selector11/1 -> Reshape11/1
  Selector16/1 -> Reshape16/1
  Reshape16/1 -> Scope16/1, Scope 16/1
  Selector18/1 -> Reshape18/1
  Reshape11/1 -> Scope11/1, Scope 11/1
  Selector10/1 -> Reshape10/1
  Reshape10/1 -> Scope10/1, Scope 10/1
  Reshape17/1 -> Scope17/1, Scope 17/1
  Selector14/1 -> Reshape14/1
  Reshape14/1 -> Scope14/1, Scope 14/1
  Reshape12/1 -> Scope12/1, Scope 12/1
  Selector13/1 -> Reshape13/1
  Gain4/1 -> Selector24/1, Selector23/1, Selector22/1, Selector20/1, Selector21/1
  Reshape23/1 -> Scope23/1, Scope 23/1
  Bus Selector2/2 -> Gain5/1  "<dh0>"
  Selector22/1 -> Reshape22/1
  Reshape29/1 -> Scope29/1, Scope 29/1
  Selector29/1 -> Reshape29/1
  Bus Selector2/1 -> Gain4/1  "<h0>"
  Reshape25/1 -> Scope25/1, Scope 25/1
  Selector25/1 -> Reshape25/1
  Gain5/1 -> Selector29/1, Selector28/1, Selector27/1, Selector25/1, Selector26/1
  Selector27/1 -> Reshape27/1
  Reshape28/1 -> Scope28/1, Scope 28/1
  Selector26/1 -> Reshape26/1
  Reshape26/1 -> Scope26/1, Scope 26/1
  Selector28/1 -> Reshape28/1
  Reshape21/1 -> Scope21/1, Scope 21/1
  Selector20/1 -> Reshape20/1
  Reshape20/1 -> Scope20/1, Scope 20/1
  Reshape27/1 -> Scope27/1, Scope 27/1
  Selector24/1 -> Reshape24/1
  Reshape24/1 -> Scope24/1, Scope 24/1
  Reshape22/1 -> Scope22/1, Scope 22/1
  Selector23/1 -> Reshape23/1
  Selector21/1 -> Reshape21/1
  Reshape32/1 -> Scope32/1, Scope 32/1
  Selector33/1 -> Reshape33/1
  Selector39/1 -> Reshape39/1
  Reshape30/1 -> Scope30/1, Scope 30/1
  Reshape31/1 -> Scope31/1, Scope 31/1
  Bus Selector3/2 -> Gain7/1  "<dh0_joint>"
  Selector36/1 -> Reshape36/1
  Selector38/1 -> Reshape38/1
  Reshape39/1 -> Scope39/1, Scope 39/1
  Selector31/1 -> Reshape31/1
  Reshape38/1 -> Scope38/1, Scope 38/1
  Reshape36/1 -> Scope36/1, Scope 36/1
  Selector32/1 -> Reshape32/1
  Reshape33/1 -> Scope33/1, Scope 33/1
  Gain6/1 -> Selector34/1, Selector33/1, Selector32/1, Selector30/1, Selector31/1
  Selector37/1 -> Reshape37/1
  Gain7/1 -> Selector39/1, Selector38/1, Selector37/1, Selector35/1, Selector36/1
  Bus Selector3/1 -> Gain6/1  "<h0_joint>"
  Reshape37/1 -> Scope37/1, Scope 37/1
  Reshape35/1 -> Scope35/1, Scope 35/1
  Selector34/1 -> Reshape34/1
  Selector35/1 -> Reshape35/1
  Selector30/1 -> Reshape30/1
  Reshape34/1 -> Scope34/1, Scope 34/1
  Reshape42/1 -> Scope42/1, Scope 42/1
  Selector43/1 -> Reshape43/1
  Selector49/1 -> Reshape49/1
  Reshape40/1 -> Scope40/1, Scope 40/1
  Reshape41/1 -> Scope41/1, Scope 41/1
  Bus Selector4/2 -> Gain9/1  "<dy>"
  Selector46/1 -> Reshape46/1
  Selector48/1 -> Reshape48/1
  Reshape49/1 -> Scope49/1, Scope 49/1
  Selector41/1 -> Reshape41/1
  Reshape48/1 -> Scope48/1, Scope 48/1
  Reshape46/1 -> Scope46/1, Scope 46/1
  Selector42/1 -> Reshape42/1
  Reshape43/1 -> Scope43/1, Scope 43/1
  Gain8/1 -> Selector44/1, Selector43/1, Selector42/1, Selector40/1, Selector41/1
  Selector47/1 -> Reshape47/1
  Gain9/1 -> Selector49/1, Selector48/1, Selector47/1, Selector45/1, Selector46/1
  Bus Selector4/1 -> Gain8/1  "<y>"
  Reshape47/1 -> Scope47/1, Scope 47/1
  Reshape45/1 -> Scope45/1, Scope 45/1
  Selector44/1 -> Reshape44/1
  Selector45/1 -> Reshape45/1
  Selector40/1 -> Reshape40/1
  Reshape44/1 -> Scope44/1, Scope 44/1
  Reshape54/1 -> Scope54/1, Scope 54/1
  Selector54/1 -> Reshape54/1
  Reshape55/1 -> Scope55/1, Scope 55/1
  Gain11/1 -> Selector59/1, Selector58/1, Selector57/1, Selector55/1, Selector56/1
  Reshape57/1 -> Scope57/1, Scope 57/1
  Selector57/1 -> Reshape57/1
  Reshape53/1 -> Scope53/1, Scope 53/1
  Bus Selector5/1 -> Gain10/1  "<y_joint>"
  Selector52/1 -> Reshape52/1
  Selector51/1 -> Reshape51/1
  Reshape58/1 -> Scope58/1, Scope 58/1
  Reshape56/1 -> Scope56/1, Scope 56/1
  Reshape59/1 -> Scope59/1, Scope 59/1
  Selector58/1 -> Reshape58/1
  Selector56/1 -> Reshape56/1
  Selector50/1 -> Reshape50/1
  Selector55/1 -> Reshape55/1
  Reshape51/1 -> Scope51/1, Scope 51/1
  Reshape50/1 -> Scope50/1, Scope 50/1
  Selector59/1 -> Reshape59/1
  Gain10/1 -> Selector54/1, Selector53/1, Selector52/1, Selector50/1, Selector51/1
  Selector53/1 -> Reshape53/1
  Reshape52/1 -> Scope52/1, Scope 52/1
  Bus Selector5/2 -> Gain11/1  "<dy_joint>"
  Bus Selector6/1 -> Gain12/1  "<hd>"
  Bus Selector6/2 -> Gain13/1  "<h0>"
  Gain12/1 -> Selector64/1, Selector65/1, Selector66/1, Selector67/1, Selector68/1, Selector69/1, Selector63/1, Selector62/1, Selector61/1, Selector60/1
  Gain13/1 -> Selector79/1, Selector78/1, Selector77/1, Selector75/1, Selector72/1, Selector70/1, Selector71/1, Selector73/1, Selector74/1, Selector76/1
  Selector60/1 -> Mux/1
  Selector70/1 -> Mux/2
  Selector61/1 -> Mux1/1
  Selector71/1 -> Mux1/2
  Selector62/1 -> Mux2/1
  Selector72/1 -> Mux2/2
  Selector63/1 -> Mux3/1
  Selector73/1 -> Mux3/2
  Selector64/1 -> Mux4/1
  Selector74/1 -> Mux4/2
  Selector65/1 -> Mux5/1
  Selector75/1 -> Mux5/2
  Selector66/1 -> Mux6/1
  Selector76/1 -> Mux6/2
  Selector67/1 -> Mux7/1
  Selector77/1 -> Mux7/2
  Selector68/1 -> Mux8/1
  Selector78/1 -> Mux8/2
  Selector69/1 -> Mux9/1
  Selector79/1 -> Mux9/2
  Reshape60/1 -> Scope60/1, Scope 60/1
  Mux/1 -> Reshape60/1
  Reshape61/1 -> Scope61/1, Scope 61/1
  Mux1/1 -> Reshape61/1
  Reshape62/1 -> Scope62/1, Scope 62/1
  Mux2/1 -> Reshape62/1
  Reshape63/1 -> Scope63/1, Scope 63/1
  Mux3/1 -> Reshape63/1
  Reshape64/1 -> Scope64/1, Scope 64/1
  Mux4/1 -> Reshape64/1
  Reshape65/1 -> Scope65/1, Scope 65/1
  Mux5/1 -> Reshape65/1
  Reshape66/1 -> Scope66/1, Scope 66/1
  Mux6/1 -> Reshape66/1
  Reshape67/1 -> Scope67/1, Scope 67/1
  Mux7/1 -> Reshape67/1
  Reshape68/1 -> Scope68/1, Scope 68/1
  Mux8/1 -> Reshape68/1
  Reshape69/1 -> Scope69/1, Scope 69/1
  Mux9/1 -> Reshape69/1
  Selector89/1 -> Mux19/1
  Selector99/1 -> Mux19/2
  Reshape77/1 -> Scope77/1, Scope 77/1
  Mux16/1 -> Reshape76/1
  Reshape71/1 -> Scope71/1, Scope 71/1
  Reshape75/1 -> Scope75/1, Scope 75/1
  Mux14/1 -> Reshape74/1
  Mux10/1 -> Reshape70/1
  Mux11/1 -> Reshape71/1
  Selector86/1 -> Mux16/1
  Selector94/1 -> Mux14/2
  Selector88/1 -> Mux18/1
  Selector91/1 -> Mux11/2
  Mux12/1 -> Reshape72/1
  Mux15/1 -> Reshape75/1
  Mux19/1 -> Reshape79/1
  Gain15/1 -> Selector99/1, Selector98/1, Selector97/1, Selector95/1, Selector92/1, Selector90/1, Selector91/1, Selector93/1, Selector94/1, Selector96/1
  Selector92/1 -> Mux12/2
  Reshape79/1 -> Scope79/1, Scope 79/1
  Selector98/1 -> Mux18/2
  Bus Selector8/2 -> Gain15/1  "<h0_joint>"
  Gain14/1 -> Selector84/1, Selector85/1, Selector86/1, Selector87/1, Selector88/1, Selector89/1, Selector83/1, Selector82/1, Selector81/1, Selector80/1
  Reshape74/1 -> Scope74/1, Scope 74/1
  Selector93/1 -> Mux13/2
  Mux13/1 -> Reshape73/1
  Reshape78/1 -> Scope78/1, Scope 78/1
  Selector87/1 -> Mux17/1
  Selector96/1 -> Mux16/2
  Selector97/1 -> Mux17/2
  Reshape73/1 -> Scope73/1, Scope 73/1
  Selector80/1 -> Mux10/1
  Selector95/1 -> Mux15/2
  Mux18/1 -> Reshape78/1
  Selector82/1 -> Mux12/1
  Selector81/1 -> Mux11/1
  Bus Selector8/1 -> Gain14/1  "<hd_joint>"
  Selector84/1 -> Mux14/1
  Mux17/1 -> Reshape77/1
  Selector90/1 -> Mux10/2
  Reshape72/1 -> Scope72/1, Scope 72/1
  Selector83/1 -> Mux13/1
  Selector85/1 -> Mux15/1
  Reshape70/1 -> Scope70/1, Scope 70/1
  Reshape76/1 -> Scope76/1, Scope 76/1
  Selector109/1 -> Mux29/1
  Selector119/1 -> Mux29/2
  Reshape87/1 -> Scope87/1, Scope 87/1
  Mux26/1 -> Reshape86/1
  Reshape81/1 -> Scope81/1, Scope 81/1
  Reshape85/1 -> Scope85/1, Scope 85/1
  Mux24/1 -> Reshape84/1
  Mux20/1 -> Reshape80/1
  Mux21/1 -> Reshape81/1
  Selector106/1 -> Mux26/1
  Selector114/1 -> Mux24/2
  Selector108/1 -> Mux28/1
  Selector111/1 -> Mux21/2
  Mux22/1 -> Reshape82/1
  Mux25/1 -> Reshape85/1
  Mux29/1 -> Reshape89/1
  Gain17/1 -> Selector119/1, Selector118/1, Selector117/1, Selector115/1, Selector112/1, Selector110/1, Selector111/1, Selector113/1, Selector114/1, Selector116/1
  Selector112/1 -> Mux22/2
  Reshape89/1 -> Scope89/1, Scope 89/1
  Selector118/1 -> Mux28/2
  Bus Selector9/2 -> Gain17/1  "<dh0>"
  Gain16/1 -> Selector104/1, Selector105/1, Selector106/1, Selector107/1, Selector108/1, Selector109/1, Selector103/1, Selector102/1, Selector101/1, Selector100/1
  Reshape84/1 -> Scope84/1, Scope 84/1
  Selector113/1 -> Mux23/2
  Mux23/1 -> Reshape83/1
  Reshape88/1 -> Scope88/1, Scope 88/1
  Selector107/1 -> Mux27/1
  Selector116/1 -> Mux26/2
  Selector117/1 -> Mux27/2
  Reshape83/1 -> Scope83/1, Scope 83/1
  Selector100/1 -> Mux20/1
  Selector115/1 -> Mux25/2
  Mux28/1 -> Reshape88/1
  Selector102/1 -> Mux22/1
  Selector101/1 -> Mux21/1
  Bus Selector9/1 -> Gain16/1  "<dhd>"
  Selector104/1 -> Mux24/1
  Mux27/1 -> Reshape87/1
  Selector110/1 -> Mux20/2
  Reshape82/1 -> Scope82/1, Scope 82/1
  Selector103/1 -> Mux23/1
  Selector105/1 -> Mux25/1
  Reshape80/1 -> Scope80/1, Scope 80/1
  Reshape86/1 -> Scope86/1, Scope 86/1
  Selector129/1 -> Mux39/1
  Selector139/1 -> Mux39/2
  Reshape97/1 -> Scope97/1, Scope 97/1
  Mux36/1 -> Reshape96/1
  Reshape91/1 -> Scope91/1, Scope 91/1
  Reshape95/1 -> Scope95/1, Scope 95/1
  Mux34/1 -> Reshape94/1
  Mux30/1 -> Reshape90/1
  Mux31/1 -> Reshape91/1
  Selector126/1 -> Mux36/1
  Selector134/1 -> Mux34/2
  Selector128/1 -> Mux38/1
  Selector131/1 -> Mux31/2
  Mux32/1 -> Reshape92/1
  Mux35/1 -> Reshape95/1
  Mux39/1 -> Reshape99/1
  Bus Selector7/1 -> Mux29/3, Mux28/3, Mux27/3, Mux26/3, Mux25/3, Mux24/3, Mux23/3, Mux22/3, Mux21/3, Mux20/3, Mux9/3, Mux8/3, Mux7/3, Mux6/3, Mux5/3, Mux4/3, Mux3/3, Mux2/3, Mux1/3, Mux/3  "<stanceLeg>"
  Gain19/1 -> Selector139/1, Selector138/1, Selector137/1, Selector135/1, Selector132/1, Selector130/1, Selector131/1, Selector133/1, Selector134/1, Selector136/1
  Selector132/1 -> Mux32/2
  Reshape99/1 -> Scope99/1, Scope 99/1
  Selector138/1 -> Mux38/2
  Bus Selector10/2 -> Gain19/1  "<dhd_joint>"
  Gain18/1 -> Selector124/1, Selector125/1, Selector126/1, Selector127/1, Selector128/1, Selector129/1, Selector123/1, Selector122/1, Selector121/1, Selector120/1
  Reshape94/1 -> Scope94/1, Scope 94/1
  Selector133/1 -> Mux33/2
  Mux33/1 -> Reshape93/1
  Reshape98/1 -> Scope98/1, Scope 98/1
  Selector127/1 -> Mux37/1
  Selector136/1 -> Mux36/2
  Selector137/1 -> Mux37/2
  Reshape93/1 -> Scope93/1, Scope 93/1
  Selector120/1 -> Mux30/1
  Selector135/1 -> Mux35/2
  Mux38/1 -> Reshape98/1
  Selector122/1 -> Mux32/1
  Selector121/1 -> Mux31/1
  Bus Selector10/1 -> Gain18/1  "<dh0_joint>"
  Selector124/1 -> Mux34/1
  Mux37/1 -> Reshape97/1
  Selector130/1 -> Mux30/2
  Reshape92/1 -> Scope92/1, Scope 92/1
  Selector123/1 -> Mux33/1
  Selector125/1 -> Mux35/1
  Reshape90/1 -> Scope90/1, Scope 90/1
  Reshape96/1 -> Scope96/1, Scope 96/1
  Bus Selector11/1 -> Mux39/3, Mux38/3, Mux37/3, Mux36/3, Mux35/3, Mux34/3, Mux33/3, Mux32/3, Mux31/3, Mux30/3, Mux19/3, Mux18/3, Mux17/3, Mux16/3, Mux15/3, Mux14/3, Mux13/3, Mux12/3, Mux11/3, Mux10/3  "<stanceLeg>"
  Selector140/1 -> Reshape100/1
  Reshape102/1 -> Scope102/1, Scope 102/1
  Selector142/1 -> Reshape102/1
  Reshape101/1 -> Scope101/1, Scope 101/1
  Selector141/1 -> Reshape101/1
  Reshape100/1 -> Scope100/1, Scope 100/1
  Reshape103/1 -> Scope103/1, Scope 103/1
  Selector143/1 -> Reshape103/1
  Reshape104/1 -> Scope104/1, Scope 104/1
  Bus Selector12/1 -> Selector144/1, Selector143/1, Selector142/1, Selector140/1, Selector141/1  "<u>"
  Selector144/1 -> Reshape104/1
  In1/1 -> Bus Selector/1, Bus Selector12/1, Bus Selector9/1, Bus Selector7/1, Bus Selector6/1, Bus Selector4/1, Bus Selector2/1, Bus Selector8/1, Bus Selector11/1, Bus Selector10/1, Bus Selector5/1, Bus Selector3/1, Bus Selector1/1, Bus Selector13/1
  Reshape105/1 -> Scope105/1, Scope 105/1
  Bus Selector13/1 -> Reshape105/1  "<torso_vx_b>"
  Reshape106/1 -> Scope106/1, Scope 106/1
  Reshape107/1 -> Scope107/1, Scope 107/1
  Reshape108/1 -> Scope108/1, Scope 108/1
  Reshape109/1 -> Scope109/1, Scope 109/1
  Reshape110/1 -> Scope110/1, Scope 110/1
  Reshape111/1 -> Scope111/1, Scope 111/1
  Bus Selector13/2 -> Reshape106/1  "<torso_vy_b>"
  Bus Selector13/3 -> Reshape107/1  "<torso_vz_b>"
  Bus Selector13/4 -> Reshape108/1  "<torso_vx_b_fil>"
  Bus Selector13/5 -> Reshape109/1  "<torso_vy_b_fil>"
  Bus Selector13/6 -> Reshape110/1  "<torso_vz_b_fil>"
  Bus Selector13/7 -> Reshape111/1  "<tg_velocity_x>"
